simulink model "progetto3cSimulink"  (R2021a)
settings: Solver=VariableStepAuto  StartTime=0.0  StopTime=10.0  RelTol=1e-3
values from neighbouring files (symbols this model uses):
  A = [0 , 1; 0 , -(bb/(Mi*Ei*Ei+Ie))-(( (Ud*Mi*Ei*Ei)/(Mi*Ei*Ei+Ie) )*2*We) ]    [Progetto3a.m]    (also in Progetto4c.m = [0, 1; ((-gg*mm*ee)*cos(pi/2))/((mm*ee*ee+Ie)), -beta/(mm*ee; ProgettoGruppoAO.m; Progetto_Ada.m = [0, 1; ((-gg*mm*ee)*cos(pi/2))/((mm*ee*ee+Ie)), -beta/(mm*ee; Prova.m = [0, 1; 0, (bb/(Mi*Ei*Ei+Ie))-(( (Ud*Mi*Ei*Ei)/(Mi*Ei*Ei+Ie) )
  B = [0; 1/(Mi*Ei*Ei+Ie)]    [Progetto3a.m]    (also in Progetto4c.m = [0;1/(mm*ee*ee + Ie)]; ProgettoGruppoAO.m; Progetto_Ada.m = [0;1/(mm*ee*ee + Ie)]; Prova.m)
  C = [0 , 1]    [Progetto3a.m]    (also in Progetto4c.m = [0, 1]; ProgettoGruppoAO.m; Progetto_Ada.m = [0, 1]; Prova.m = [0, 1])
  den_r = d_r{1}    [Progetto3a.m]    (also in Progetto4c.m; ProgettoGruppoAO.m; Progetto_Ada.m; Prova.m)
  num_r = n_r{1}    [Progetto3a.m]    (also in Progetto4c.m; ProgettoGruppoAO.m; Progetto_Ada.m; Prova.m)
  omega_n = 100    [Progetto3a.m]    (also in Progetto4c.m = 120; ProgettoGruppoAO.m; Progetto_Ada.m = 120; Prova.m)
  W = 5    [Progetto3a.m]    (also in Progetto4c.m = 4; ProgettoGruppoAO.m; Progetto_Ada.m = 4; Prova.m)
  x0 = [0,We]    [Progetto3a.m]    (also in Progetto4c.m = [0;0]; ProgettoGruppoAO.m = [teta_e,We]; Progetto_Ada.m = [0;0]; Prova.m = [teta_e,We])
settings Model: Creator=Giacomo  LastModifiedBy=Giacomo

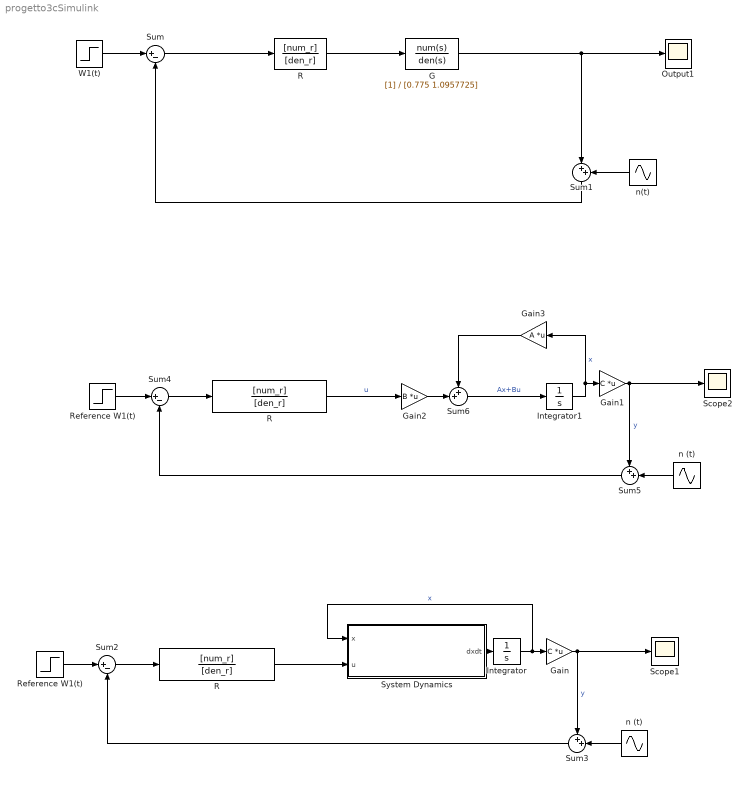
== system progetto3cSimulink ==
  G : TransferFcn  Denominator=[0.775 1.0957725]
  Gain : Gain  Gain=C  Multiplication=Matrix(K*u)
  Gain1 : Gain  Gain=C  Multiplication=Matrix(K*u)
  Gain2 : Gain  Gain=B  Multiplication=Matrix(K*u)
  Gain3 : Gain  Gain=A  Multiplication=Matrix(K*u)
  Integrator : Integrator  InitialCondition=x0
  Integrator1 : Integrator  InitialCondition=x0
  Output1 : Scope
  R : TransferFcn  Numerator=[num_r]  Denominator=[den_r]
  "R " : TransferFcn  Numerator=[num_r]  Denominator=[den_r]
  "R " : TransferFcn  Numerator=[num_r]  Denominator=[den_r]
  "Reference W1(t) " : Step  After=W  SampleTime=0
  "Reference W1(t) " : Step  After=W  SampleTime=0
  Scope1 : Scope
  Scope2 : Scope
  Sum : Sum  Inputs=|+-
  Sum1 : Sum  Inputs=|++
  Sum2 : Sum  Inputs=|+-
  Sum3 : Sum  Inputs=++|
  Sum4 : Sum  Inputs=|+-
  Sum5 : Sum  Inputs=++|
  Sum6 : Sum  Inputs=++|
  System Dynamics : MATLAB Function  TreatAsAtomicUnit=on
  W1(t) : Step  After=W  SampleTime=0
  n (t) : Sin  Amplitude=0.02  Frequency=omega_n  SampleTime=0
  "n (t) " : Sin  Amplitude=0.02  Frequency=omega_n  SampleTime=0
  n(t) : Sin  Amplitude=0.02  Frequency=omega_n  SampleTime=0  VectorParams1D=off
  wires:
  Sum1/1 -> Sum/2
  W1(t)/1 -> Sum/1
  G/1 -> Output1/1, Sum1/1
  R/1 -> G/1
  n(t)/1 -> Sum1/2
  Sum/1 -> R/1
  Sum6/1 -> Integrator1/1  "Ax+Bu"
  Gain3/1 -> Sum6/1
  "Reference W1(t) "/1 -> Sum4/1
  Gain2/1 -> Sum6/2
  "n (t) "/1 -> Sum5/2
  Sum4/1 -> "R "/1
  Gain1/1 -> Sum5/1, Scope2/1  "y"
  Integrator1/1 -> Gain1/1, Gain3/1  "x"
  "R "/1 -> Gain2/1  "u"
  Sum5/1 -> Sum4/2
  n (t)/1 -> Sum3/2
  "Reference W1(t) "/1 -> Sum2/1
  Sum3/1 -> Sum2/2
  System Dynamics/1(dxdt) -> Integrator/1
  Gain/1 -> Scope1/1, Sum3/1  "y"
  Integrator/1 -> System Dynamics/1(x), Gain/1  "x"
  Sum2/1 -> "R "/1
  "R "/1 -> System Dynamics/2(u)

== matlab function progetto3cSimulink/System Dynamics ==
  data: x input; u input; dxdt output
function dxdt = systemDynamics(x,u)
%tau
Ue=-477.06;
dx1dt=x(2);
dx2dt=( -bb*x(2)- (Ud*Mi*Ei*Ei*x(2)*x(2) )+ Ue ) / dist_mas_iner;
%dxdt = [dx1dt; dx2dt; dx3dt;...;dxndt];
dxdt = [dx1dt; dx2dt];
